simulink model "untitled1"  (R2023b)
settings: Solver=VariableStepAuto  StartTime=0.0  StopTime=10.0  RelTol=1e-3
settings Model: Creator=didad  LastModifiedBy=didad

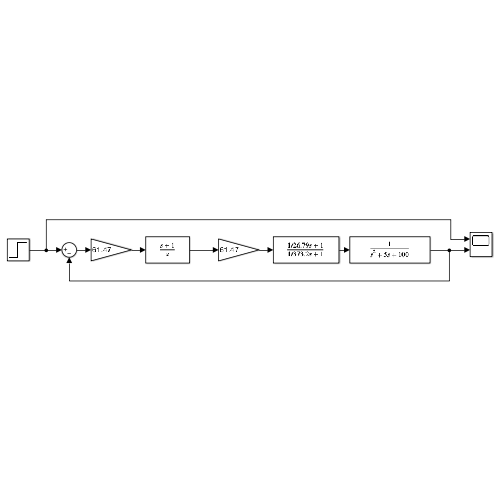
[thumbnail: Simulink's stored preview of the top-level diagram]
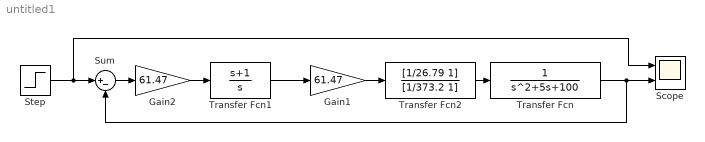
== system untitled1 ==
  Gain1 : Gain  Gain=61.47
  Gain2 : Gain  Gain=61.47
  Scope : Scope  NumInputPorts=2
  Step : Step  SampleTime=0
  Sum : Sum  Inputs=|+-
  Transfer Fcn : TransferFcn  Denominator=[1 5 100]
  Transfer Fcn1 : TransferFcn  Numerator=[1 1]  Denominator=[1 0]
  Transfer Fcn2 : TransferFcn  Numerator=[1/26.79 1]  Denominator=[1/373.2 1]
  wires:
  Sum/1 -> Gain2/1
  Step/1 -> Sum/1, Scope/1
  Transfer Fcn/1 -> Scope/2, Sum/2
  Gain2/1 -> Transfer Fcn1/1
  Transfer Fcn2/1 -> Transfer Fcn/1
  Transfer Fcn1/1 -> Gain1/1
  Gain1/1 -> Transfer Fcn2/1
